simulink model "PVFarmDistributionSystem"  (R2022b)
settings: Solver=FixedStepDiscrete  StartTime=0.0  StopTime=0.6  FixedStep=Ts_Power  RelTol=1e-4
PreLoadFcn:
  | Ts_Power=1e-6;
  | Ts=25e-6;
undefined symbols (not defined in the file): D1, Delta, DiscIntNeverNeededParam, Ion, Lithium
libraries: spsSeriesRLCBranchLib x10, simulink x8, spsMeanLib x5, spsFirstOrderFilterLib x4, spsStairGeneratorLib x4, spsThreePhaseVIMeasurementLib x3, spsPWMGeneratorDCDCLib x3, spsThreePhaseTransformerTwoWindingsLib x2, spsThreePhaseParallelRLCLoadLib x2, spsThreePhasePISectionLineLib x2, spsBoostConverterLib x2, spsPowerPositiveSequenceLib x2
(part 1 of 2)
settings Model: SimulationMode=accelerator  Creator=The MathWorks, Inc.  LastModifiedBy=刘明炜
settings SolverCC: AlgebraicLoopSolver=TrustRegion
settings DataIOCC: SaveOutput=off  SignalLogging=off  DSMLogging=off  SaveTime=off  ReturnWorkspaceOutputs=off
settings OptimizationCC: ReuseModelBlockBuffer=on
settings DebuggingCC: UnconnectedInputMsg=warning  UnconnectedOutputMsg=warning  UnconnectedLineMsg=warning  ArithmeticOperatorsInVariantConditions=warning
settings ModelReferenceCC: EnableRefExpFcnMdlSchedulingChecks=on
settings SFSimCC: CustomCodeUndefinedFunction=UseInterfaceOnly

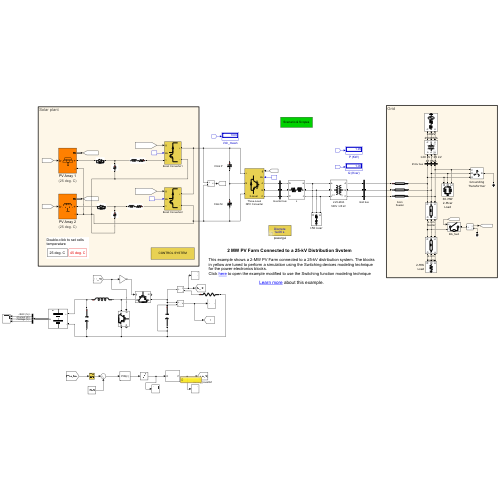
[thumbnail: Simulink's stored preview of the top-level diagram]
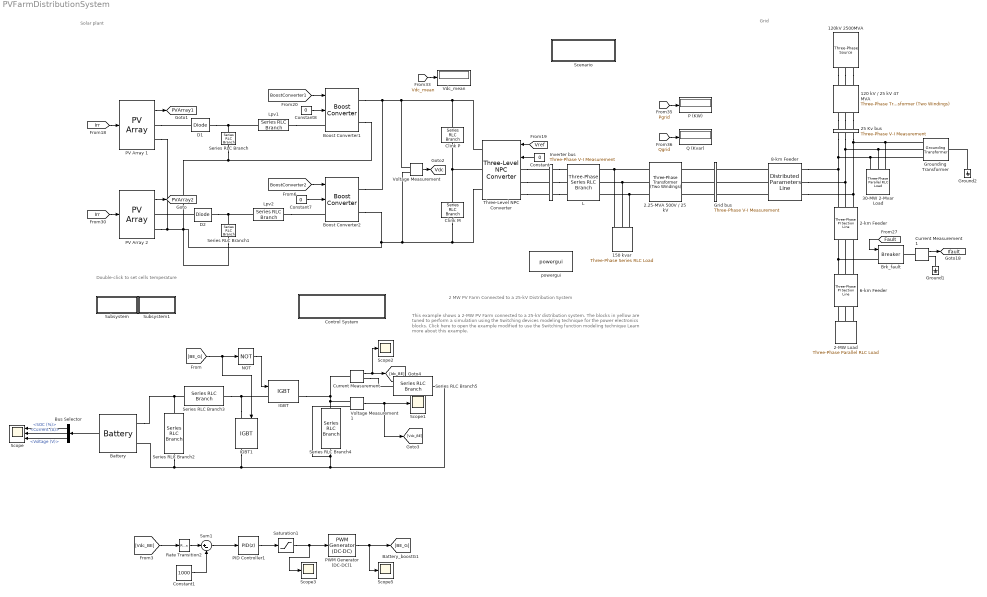
== system PVFarmDistributionSystem ==
  note: Grid
  note: Solar plant
  note: Double-click to set cells temperature
  note: 2 MW PV Farm Connected to a 25-kV Distribution System
  note: This example shows a 2-MW PV Farm connected to a 25-kV distribution system. The blocks in yellow are tuned to perform a simulation using the Switching devices modeling technique for the power electronics blocks.
      | Click here to open the example modified to use the Switching function modeling technique
      |
      | Learn more about this example.
  120 kV / 25 kV 47 MVA : spsThreePhaseTransformerTwoWindingsLib/Three-Phase Transformer (Two Windings)  Winding1Connection=Yg  Winding2Connection=Delta (D1)  CoreType=Three single-phase transformers  SetSaturation=off  Hysteresis=off  DataFile='basic_model'  SetInitialFlux=off  Measurements=None  UNITS=pu  NominalPower=[47e6 50 ]  Winding1="[ 120e3  0.08/30   0.08 ]"  Winding2="[ 25e3 0.08/30  0.08]"  Rm=500  Lm=500  L0=0.5  Saturation="[ 0,0  ;  0.005,1.2  ;  1.0,1.4 ]"  InitialFluxes=[ 0.8 , -0.8 , 0.7 ]  BreakLoop=off  DiscreteSolver=Trapezoidal iterative  DataType=off  TransfoNumber=0
  120kV 2500MVA : spsThreePhaseSourceLib/Three-Phase Source  InternalConnection=Yg  VoltagePhases=off  Voltage=120e3*1.02  PhaseAngle=0  Voltage_phases=[25e3 25e3 25e3]/sqrt(3)  PhaseAngles_phases=[0 -120 +120]  Frequency=50  NonIdealSource=on  SpecifyImpedance=on  Resistance=0.8929  Inductance=16.58e-3  ShortCircuitLevel=2500e6  BaseVoltage=120e3  XRratio=7  BusType=swing  Pref=0  Qref=0  Prefabc=[10e3, 10e3, 10e3]  Qrefabc=[0, 0, 0]  Qmin=-inf  Qmax=inf
  150 kvar : spsThreePhaseSeriesRLCLoadLib/Three-Phase Series RLC Load  LConnTagsString=A|B|C  Configuration=Y (grounded)  NominalVoltage=500  Vabc=[1e3 1e3 1e3]  Vabcp=[1e3 1e3 1e3]  NominalFrequency=50  UnbalancedPower=off  ActivePower=150e3/50  InductivePower=0  CapacitivePower=150e3  Pabc=[10e3 9e3 11e3]  QLabc=[100 90 110]  QCabc=[100 90 110]  Pabcp=[10e3 9e3 11e3]  QLabcp=[100 90 110]  QCabcp=[100 90 110]  Measurements=None  LoadType=constant Z
  2-MW Load : spsThreePhaseParallelRLCLoadLib/Three-Phase Parallel RLC Load  LConnTagsString=A|B|C  Configuration=Y (grounded)  NominalVoltage=25e3  Vabc=[1e3 1e3 1e3]  Vabcp=[1e3 1e3 1e3]  NominalFrequency=50  UnbalancedPower=off  ActivePower=2e6  InductivePower=0  CapacitivePower=0  Pabc=[10e3 9e3 11e3]  QLabc=[100 90 110]  QCabc=[100 90 110]  Pabcp=[10e3 9e3 11e3]  QLabcp=[100 90 110]  QCabcp=[100 90 110]  Measurements=None  LoadType=constant Z
  2-km Feeder : spsThreePhasePISectionLineLib/Three-Phase PI Section Line  LConnTagsString=a|b|c  RConnTagsString=A|B|C  Length=2  Frequency=50  Resistances=[0.1153 0.413]  Inductances=[1.05e-3 3.32e-3]  Capacitances=[11.33e-009 5.01e-009]
  2.25-MVA 500V / 25 kV : spsThreePhaseTransformerTwoWindingsLib/Three-Phase Transformer (Two Windings)  Winding1Connection=Yg  Winding2Connection=Delta (D1)  CoreType=Three single-phase transformers  SetSaturation=off  Hysteresis=off  DataFile='hysteresis'  SetInitialFlux=off  Measurements=None  UNITS=pu  NominalPower=[2.25e6 , 50 ]  Winding1=[ 25e3 , 0.001 , 0.03 ]  Winding2=[500 , 0.001 , 0.03 ]  Rm=200  Lm=200  L0=0.5  Saturation=[ 0,0 ; 0.0024,1.2 ; 1.0,1.52 ]  InitialFluxes=[ 0.8 , -0.8 , 0.7 ]  BreakLoop=off  DiscreteSolver=Trapezoidal iterative  DataType=off  TransfoNumber=0
  25 Kv bus : spsThreePhaseVIMeasurementLib/Three-Phase V-I Measurement  VoltageMeasurement=phase-to-ground  SetLabelV=on  LabelV=Vabc25kV  Vpu=off  VpuLL=off  CurrentMeasurement=yes  SetLabelI=on  LabelI=Iabc25kV  Ipu=off  Pbase=100e6  Vbase=500e3  OutputType=Complex  PhasorSimulation=off  PSBequivalent=0
  30-MW 2-Mvar Load : spsThreePhaseParallelRLCLoadLib/Three-Phase Parallel RLC Load  LConnTagsString=A|B|C  Configuration=Y (grounded)  NominalVoltage=25e3  Vabc=[1e3 1e3 1e3]  Vabcp=[1e3 1e3 1e3]  NominalFrequency=50  UnbalancedPower=off  ActivePower=30e6  InductivePower=2e6  CapacitivePower=0  Pabc=[10e3 9e3 11e3]  QLabc=[100 90 110]  QCabc=[100 90 110]  Pabcp=[10e3 9e3 11e3]  QLabcp=[100 90 110]  QCabcp=[100 90 110]  Measurements=None  LoadType=constant Z
  6-km Feeder : spsThreePhasePISectionLineLib/Three-Phase PI Section Line  LConnTagsString=a|b|c  RConnTagsString=A|B|C  Length=6  Frequency=50  Resistances=[0.1153 0.413]  Inductances=[1.05e-3 3.32e-3]  Capacitances=[11.33e-009 5.01e-009]
  8-km Feeder : spsDistributedParametersLineLib/Distributed Parameters Line  Phases=3  Length=8  Frequency=50  Resistance=[0.1153 0.413]  Inductance=[1.05e-3 3.32e-3]  Capacitance=[11.33e-009 5.01e-009]  x1=[-3.3e-05 -0.0265033347341034 -3248.46958209552 -24803.9467011839;-3.2e-05 -0.0265134091291118 -3240.67704414589 -24804.9660112368;-3.1e-05 -0.0265234809073516 -3232.88418635427 -24805.9828731378;-3e-05 -0.0265335500678288 -3225.09100948977 -24806.9972867864;-2.9e-05 -0.0265436166095496 -3217.29751432154 -24808.0092520825;-2.8e-05 -0.0265536805315205 -3209.50370161879 -24809.0187689262;-2.7e-05 -0.0265637418327481 -3201.70957215071 -24810.025837218;-2.6e-05 -0.0265738005122396 -3193.91512668657 -24811.0304568584;-2.5e-05 -0.026583856569002 -3186.12036599565 -24812.0326277483;-2.4e-05 -0.0265939100020431 -3178.32529084725 -24813.0323497887;-2.3e-05 -0.0266039608103704 -3170.52990201072 -24814.029622881;-2.2e-05 -0.0266140089929921 -3162.73420025543 -24815.0244469268;-2.1e-05 -0.0266240545489164 -3154.9381863508 -24816.0168218278;-2e-05 -0.0266340974771518 -3147.14186106624 -24817.0067474862;-1.9e-05 -0.0266441377767072 -3139.34522517124 -24817.9942238042;-1.8e-05 -0.0266541754465917 -3131.54827943529 -24818.9792506844;-1.7e-05 -0.0266642104858145 -3123.75102462791 -24819.9618280295;-1.6e-05 -0.0266742428933852 -3115.95346151867 -24820.9419557426;-1.5e-05 -0.0266842726683137 -3108.15559087715 -24821.9196337269;-1.4e-05 -0.0266942998096101 -3100.35741347297 -24822.894861886;-1.3e-05 -0.0267043243162847 -3092.55893007578 -24823.8676401236;-1.2e-05 -0.0267143461873481 -3084.76014145526 -24824.8379683437;-1.1e-05 -0.0267243654218113 -3076.96104838112 -24825.8058464505;-1e-05 -0.0267343820186854 -3069.1616516231 -24826.7712743485;-9e-06 -0.0267443959769817 -3061.36195195097 -24827.7342519424;-8e-06 -0.026754407295712 -3053.56195013453 -24828.6947791371;-7e-06 -0.0267644159738881 -3045.76164694361 -24829.652855838;-6e-06 -0.0267744220105223 -3037.96104314806 -24830.6084819503;-5e-06 -0.026784425404627 -3030.16013951778 -24831.5616573798;-4e-06 -0.0267944261552148 -3022.35893682268 -24832.5123820325;-3e-06 -0.0268044242612989 -3014.55743583272 -24833.4606558144;-2e-06 -0.0268144197218923 -3006.75563731786 -24834.406478632;-1e-06 -0.0268244125360086 -2998.95354204812 -24835.349850392]  x2=[-3.3e-05 -0.0341174630392466 -3239.57935848666 -24789.8574696466;-3.2e-05 -0.0341341517787849 -3231.79124723035 -24790.8739874471;-3.1e-05 -0.0341508371494174 -3224.00281700904 -24791.8880584864;-3e-05 -0.0341675191494974 -3216.2140685914 -24792.8996826644;-2.9e-05 -0.0341841977773784 -3208.42500274616 -24793.9088598814;-2.8e-05 -0.0342008730314144 -3200.63562024207 -24794.9155900376;-2.7e-05 -0.0342175449099596 -3192.8459218479 -24795.9198730338;-2.6e-05 -0.0342342134113685 -3185.05590833248 -24796.9217087708;-2.5e-05 -0.0342508785339959 -3177.26558046464 -24797.9210971498;-2.4e-05 -0.0342675402761972 -3169.47493901326 -24798.9180380721;-2.3e-05 -0.0342841986363279 -3161.68398474725 -24799.9125314392;-2.2e-05 -0.0343008536127438 -3153.89271843553 -24800.9045771532;-2.1e-05 -0.0343175052038011 -3146.10114084709 -24801.894175116;-2e-05 -0.0343341534078565 -3138.30925275091 -24802.8813252299;-1.9e-05 -0.0343507982232668 -3130.51705491602 -24803.8660273977;-1.8e-05 -0.0343674396483892 -3122.72454811149 -24804.848281522;-1.7e-05 -0.0343840776815814 -3114.9317331064 -24805.8280875059;-1.6e-05 -0.0344007123212011 -3107.13861066987 -24806.8054452527;-1.5e-05 -0.0344173435656066 -3099.34518157106 -24807.780354666;-1.4e-05 -0.0344339714131565 -3091.55144657914 -24808.7528156495;-1.3e-05 -0.0344505958622096 -3083.75740646333 -24809.7228281073;-1.2e-05 -0.0344672169111253 -3075.96306199286 -24810.6903919437;-1.1e-05 -0.034483834558263 -3068.16841393701 -24811.655507063;-1e-05 -0.0345004488019827 -3060.37346306507 -24812.6181733701;-9e-06 -0.0345170596406447 -3052.57821014639 -24813.57839077;-8e-06 -0.0345336670726094 -3044.78265595031 -24814.5361591679;-7e-06 -0.0345502710962378 -3036.98680124624 -24815.4914784692;-6e-06 -0.0345668717098912 -3029.19064680358 -24816.4443485798;-5e-06 -0.0345834689119311 -3021.39419339179 -24817.3947694054;-4e-06 -0.0346000627007194 -3013.59744178035 -24818.3427408524;-3e-06 -0.0346166530746185 -3005.80039273877 -24819.2882628272;-2e-06 -0.0346332400319909 -2998.00304703658 -24820.2313352364;-1e-06 -0.0346498235711995 -2990.20540544335 -24821.171957987]  x3=[-3.3e-05 0.0018330109452432 -5.20094376290719 -82.5841573333767;-3.2e-05 0.00183248033431178 -5.17499896715227 -82.5857871710245;-3.1e-05 0.00183194954252181 -5.14905366064543 -82.587408857782;-3e-05 0.00183141856992567 -5.12310784594737 -82.589022393489;-2.9e-05 0.00183088741657575 -5.09716152561884 -82.5906277779862;-2.8e-05 0.0018303560825245 -5.07121470222063 -82.5922250111153;-2.7e-05 0.00182982456782434 -5.0452673783136 -82.5938140927186;-2.6e-05 0.00182929287252774 -5.01931955645864 -82.5953950226393;-2.5e-05 0.00182876099668717 -4.9933712392167 -82.5969678007212;-2.4e-05 0.00182822894035512 -4.96742242914877 -82.5985324268093;-2.3e-05 0.00182769670358412 -4.94147312881591 -82.600088900749;-2.2e-05 0.00182716428642668 -4.9155233407792 -82.6016372223868;-2.1e-05 0.00182663168893535 -4.88957306759979 -82.6031773915699;-2e-05 0.0018260989111627 -4.86362231183886 -82.6047094081462;-1.9e-05 0.00182556595316132 -4.83767107605766 -82.6062332719645;-1.8e-05 0.0018250328149838 -4.81171936281746 -82.6077489828744;-1.7e-05 0.00182449949668277 -4.7857671746796 -82.6092565407264;-1.6e-05 0.00182396599831085 -4.75981451420545 -82.6107559453717;-1.5e-05 0.0018234323199207 -4.73386138395645 -82.6122471966622;-1.4e-05 0.00182289846156501 -4.70790778649406 -82.6137302944507;-1.3e-05 0.00182236442329644 -4.6819537243798 -82.615205238591;-1.2e-05 0.00182183020516772 -4.65599920017523 -82.6166720289374;-1.1e-05 0.00182129580723156 -4.63004421644197 -82.6181306653452;-1e-05 0.00182076122954072 -4.60408877574165 -82.6195811476704;-9e-06 0.00182022647214794 -4.578132880636 -82.6210234757698;-8e-06 0.00181969153510602 -4.55217653368674 -82.6224576495012;-7e-06 0.00181915641846774 -4.52621973745568 -82.6238836687229;-6e-06 0.00181862112228592 -4.50026249450463 -82.6253015332942;-5e-06 0.00181808564661339 -4.47430480739548 -82.6267112430751;-4e-06 0.00181754999150301 -4.44834667869016 -82.6281127979266;-3e-06 0.00181701415700763 -4.42238811095061 -82.6295061977104;-2e-06 0.00181647814318014 -4.39642910673886 -82.6308914422888;-1e-06 0.00181594195007344 -4.37046966861695 -82.6322685315251]  x4=[-3.3e-05 -0.00190671763640625 -16.7682219944814 -79.863855689428;-3.2e-05 -0.00190621992184286 -16.743131236574 -79.8691196346437;-3.1e-05 -0.0019057220191431 -16.7180388261858 -79.8743756970934;-3e-05 -0.00190522392835613 -16.6929447657932 -79.8796238762582;-2.9e-05 -0.00190472564953108 -16.6678490578731 -79.8848641716203;-2.8e-05 -0.00190422718271716 -16.6427517049023 -79.8900965826623;-2.7e-05 -0.00190372852796354 -16.6176527093577 -79.8953211088679;-2.6e-05 -0.00190322968531946 -16.5925520737165 -79.9005377497214;-2.5e-05 -0.00190273065483413 -16.5674498004561 -79.905746504708;-2.4e-05 -0.00190223143655682 -16.542345892054 -79.9109473733137;-2.3e-05 -0.00190173203053679 -16.5172403509877 -79.916140355025;-2.2e-05 -0.00190123243682333 -16.4921331797352 -79.9213254493294;-2.1e-05 -0.00190073265546575 -16.4670243807744 -79.9265026557153;-2e-05 -0.00190023268651339 -16.4419139565835 -79.9316719736716;-1.9e-05 -0.00189973253001557 -16.4168019096407 -79.9368334026881;-1.8e-05 -0.00189923218602167 -16.3916882424245 -79.9419869422555;-1.7e-05 -0.00189873165458107 -16.3665729574136 -79.9471325918651;-1.6e-05 -0.00189823093574317 -16.3414560570866 -79.9522703510091;-1.5e-05 -0.00189773002955739 -16.3163375439227 -79.9574002191803;-1.4e-05 -0.00189722893607316 -16.2912174204007 -79.9625221958725;-1.3e-05 -0.00189672765533994 -16.2660956890001 -79.9676362805801;-1.2e-05 -0.00189622618740721 -16.2409723522001 -79.9727424727985;-1.1e-05 -0.00189572453232445 -16.2158474124805 -79.9778407720236;-1e-05 -0.00189522269014119 -16.1907208723209 -79.9829311777523;-9e-06 -0.00189472066090694 -16.1655927342012 -79.9880136894821;-8e-06 -0.00189421844467126 -16.1404630006014 -79.9930883067115;-7e-06 -0.00189371604148372 -16.1153316740019 -79.9981550289396;-6e-06 -0.0018932134513939 -16.0901987568828 -80.0032138556663;-5e-06 -0.0018927106744514 -16.0650642517248 -80.0082647863924;-4e-06 -0.00189220771070584 -16.0399281610085 -80.0133078206194;-3e-06 -0.00189170456020688 -16.0147904872148 -80.0183429578494;-2e-06 -0.00189120122300415 -15.9896512328247 -80.0233701975856;-1e-06 -0.00189069769914735 -15.9645104003192 -80.0283895393318]  x5=3.26270562570392e-05  V1=ones(3,3)  V2=ones(3,3)  I1=ones(3,3)  I2=ones(3,3)  nHarmo=1  Measurements=None  Decoupling=off  VsMag0=0  VrMag0=0  VsAngle0=0  VrAngle0=0  IsMag0=0  IrMag0=0  IsAngle0=0  IrAngle0=0
      settings: LibrarySourceBlock=sps_lib/Power Grid Elements/Distributed Parameters Line
  Battery : spsBatteryLib/Battery  BatType=Lithium-Ion  ShowTempParam=off  ThermalPreset=no  ShowAgeParam=off  NomV=300  NomQ=100  SOC=70  Batt_Tr=1  PresetModel=on  MaxQ=100  MinV=225  FullV=349.1961  Dis_rate=43.4783  R=0.03  Normal_OP=90.4348  expZone="[324.1158      4.913043]"  current=[6.5 13 32.5]  Units=Time  Tci=20  NomT=20  T2=-30  MaxQ2=4.8  FullV2=7.1  Normal_OP2=5.655  expZone2="[6.58           1]"  Rca=0.6  ti=2000  Dp=0  Neq0=0  Tsim=1e6  Ta1=25  Qeol=5.4*0.9  Reol=0.013333*1.2  Char_age=[2.3478, 3]  Dis_age=[2.3478, 10]  N1=1500  N2=10500  N3=1000  N4=1400  Ta2=45  N5=950
  Boost Converter1 : spsBoostConverterLib/Boost Converter  ModelType=Switching devices  Ron=1e-4  Rs=1e6  Cs=inf  Vforward=[0,0]  Ron_Diode=1e-4  Rs_Diode=1e6  Cs_Diode=inf  Vf_Diode=0  Rs_CurrentSource=inf  Ron_ACsource=1e-3
      settings: LibrarySourceBlock=sps_lib/Power Electronics/Boost Converter
  Boost Converter2 : spsBoostConverterLib/Boost Converter  ModelType=Switching devices  Ron=1e-4  Rs=1e6  Cs=inf  Vforward=[0,0]  Ron_Diode=1e-4  Rs_Diode=1e6  Cs_Diode=inf  Vf_Diode=0  Rs_CurrentSource=inf  Ron_ACsource=1e-3
      settings: LibrarySourceBlock=sps_lib/Power Electronics/Boost Converter
  Brk_fault : spsBreakerLib/Breaker  InitialState=0  SwitchingTimes="[30/60  42/60]*999"  External=on  BreakerResistance=0.2  SnubberResistance=1e6  SnubberCapacitance=inf  Measurements=None  MoreParameters=on  NoBreakLoop=off
  Bus Selector : BusSelector  OutputSignals=SOC (%),Current (A),Voltage (V)
  Clink M : spsSeriesRLCBranchLib/Series RLC Branch  LConnTagsString=__new0  RConnTagsString=__new0  BranchType=C  Resistance=1e-6  Inductance=1e-3  SetiL0=off  InitialCurrent=0  Capacitance=150e-3  Setx0=on  InitialVoltage=500  Measurements=None
  Clink P : spsSeriesRLCBranchLib/Series RLC Branch  LConnTagsString=__new0  RConnTagsString=__new0  BranchType=C  Resistance=1e-6  Inductance=1e-3  SetiL0=off  InitialCurrent=0  Capacitance=150e-3  Setx0=on  InitialVoltage=500  Measurements=None
  Constant : Constant  Value=0  SampleTime=Ts
  Constant1 : Constant  Value=1000
  Constant7 : Constant  Value=0  SampleTime=Ts
  Constant8 : Constant  Value=0  SampleTime=Ts
  Control System : Subsystem
      mask Display: disp('CONTROL SYSTEM')
  Current Measurement : spsCurrentMeasurementLib/Current Measurement  PhasorSimulation=off  OutputType=Complex  PSBequivalent=0
  Current Measurement1 : spsCurrentMeasurementLib/Current Measurement  PhasorSimulation=off  OutputType=Complex  PSBequivalent=0
  D1 : spsDiodeLib/Diode  Ron=1e-4  Lon=0  Vf=0  IC=0  UseSnubber=0  Rs=1e6  Cs=inf  Measurements=off
  D2 : spsDiodeLib/Diode  Ron=1e-4  Lon=0  Vf=0  IC=0  UseSnubber=0  Rs=1e6  Cs=inf  Measurements=off
  Grid bus : spsThreePhaseVIMeasurementLib/Three-Phase V-I Measurement  VoltageMeasurement=phase-to-ground  SetLabelV=on  LabelV=Vgrid  Vpu=off  VpuLL=off  CurrentMeasurement=yes  SetLabelI=on  LabelI=Igrid  Ipu=off  Pbase=100e6  Vbase=500e3  OutputType=Magnitude  PhasorSimulation=off  PSBequivalent=0
  Ground1 : spsGroundLib/Ground  LConnTagsString=a
  Ground2 : spsGroundLib/Ground  LConnTagsString=a
  Grounding Transformer : spsGroundingTransformerLib/Grounding Transformer   UNITS=SI  NominalPower="[3e6   50]"  NominalVoltage=25e3  ZeroSequenceImpedance_pu=[0.0012 0.036]  MagnetizationBranch_pu=[500 500]  ZeroSequenceImpedance_SI=[0.25 7.5]  MagnetizationBranch_SI=[1.0417e+05 1.0417e+05]  Measurements=None
      settings: LibrarySourceBlock=|
      | sps_lib/Power Grid Elements/Grounding
      | Transformer
  IGBT : spsIGBTLib/IGBT  Ron=0.001  Lon=0  Vf=1  Tf=1e-6  Tt=2e-6  IC=0  Rs=1e5  Cs=inf  Measurements=on
  IGBT1 : spsIGBTLib/IGBT  Ron=0.001  Lon=0  Vf=1  Tf=1e-6  Tt=2e-6  IC=0  Rs=1e5  Cs=inf  Measurements=on
  Inverter bus : spsThreePhaseVIMeasurementLib/Three-Phase V-I Measurement  VoltageMeasurement=phase-to-phase  SetLabelV=on  LabelV=Vinv  Vpu=off  VpuLL=off  CurrentMeasurement=no  SetLabelI=off  LabelI=Iabc_B1  Ipu=off  Pbase=100e6  Vbase=500e3  OutputType=Magnitude  PhasorSimulation=off  PSBequivalent=0
  L : spsThreePhaseSeriesRLCBranchLib/Three-Phase Series RLC Branch  LConnTagsString=A|B|C  RConnTagsString=A|B|C  BranchType=RL  Resistance=1e-3  Inductance=44.2e-6  Capacitance=inf  Measurements=None
  Lpv1 : spsSeriesRLCBranchLib/Series RLC Branch  LConnTagsString=__new0  RConnTagsString=__new0  BranchType=RL  Resistance=1e-3  Inductance=1e-3  SetiL0=off  InitialCurrent=0  Capacitance=120e-3  Setx0=off  InitialVoltage=0  Measurements=None
  Lpv2 : spsSeriesRLCBranchLib/Series RLC Branch  LConnTagsString=__new0  RConnTagsString=__new0  BranchType=RL  Resistance=1e-3  Inductance=1e-3  SetiL0=off  InitialCurrent=0  Capacitance=120e-3  Setx0=off  InitialVoltage=0  Measurements=None
  NOT : Logic  Operator=NOT  IconShape=distinctive  AllPortsSameDT=off  OutDataTypeStr=boolean
  P (KW) : Display
      settings: Format=bank  Decimation=200
  PID Controller1 : slpidlib/PID Controller  Controller=PID  Form=Parallel  TimeDomain=Discrete-time  UseExternalTs=off  SampleTime=-1  IntegratorMethod=Forward Euler  FilterMethod=Forward Euler  ControllerParametersSource=internal  P=1  I=1  UseKiTs=off  D=0  N=100  UseFilter=on  TunerSelectOption=Transfer Function Based (PID Tuner App)  InitialConditionSource=internal  InitialConditionForIntegrator=0  InitialConditionForFilter=0  DifferentiatorICPrevScaledInput=0  ExternalReset=none  TrackingMode=off  Kt=1  LimitOutput=off  SatLimitsSource=internal  UpperSaturationLimit=0.99  LowerSaturationLimit=0.1  LinearizeAsGain=on  AntiWindupMode=none  Kb=1  LimitIntegrator=off  UpperIntegratorSaturationLimit=inf  LowerIntegratorSaturationLimit=-inf  POutMin=[]  POutMax=[]  IOutMin=[]  IOutMax=[]  DOutMin=[]  DOutMax=[]  NOutMin=[]  NOutMax=[]  SumOutMin=[]  SumOutMax=[]  SaturationOutMin=[]  SaturationOutMax=[]  PParamMin=[]  PParamMax=[]  IParamMin=[]  IParamMax=[]  DParamMin=[]  DParamMax=[]  NParamMin=[]  NParamMax=[]  KbParamMin=[]  KbParamMax=[]  KtParamMin=[]  KtParamMax=[]  KbOutMin=[]  KbOutMax=[]  KtOutMin=[]  KtOutMax=[]  IntegratorOutMin=[]  IntegratorOutMax=[]  FilterOutMin=[]  FilterOutMax=[]  SumI1OutMin=[]  SumI1OutMax=[]  SumI2OutMin=[]  SumI2OutMax=[]  SumI3OutMin=[]  SumI3OutMax=[]  SumI4OutMin=[]  SumI4OutMax=[]  SumDOutMin=[]  SumDOutMax=[]  DifferentiatorOutMin=[]  DifferentiatorOutMax=[]  FilterDiffOutCoefMin=[]  FilterDiffOutCoefMax=[]  ReciprocalOutMin=[]  ReciprocalOutMax=[]  SumDenOutMin=[]  SumDenOutMax=[]  SumNumOutMin=[]  SumNumOutMax=[]  DivideOutMin=[]  DivideOutMax=[]  UdiffTsProdOutMin=[]  UdiffTsProdOutMax=[]  NTsProdOutMin=[]  NTsProdOutMax=[]  UintegralTsProdOutMin=[]  UintegralTsProdOutMax=[]  UngainTsProdOutMin=[]  UngainTsProdOutMax=[]  ClampingZeroOutDataTypeStr=Inherit: Inherit via back propagation  ClampingZeroOutMin=[]  ClampingZeroOutMax=[]  FilterDenConstantOutDataTypeStr=Inherit: Inherit via back propagation  FilterDenConstantOutMin=[]  FilterDenConstantOutMax=[]  PCopyOutDataTypeStr=Inherit: Inherit via back propagation  PCopyOutMin=[]  PCopyOutMax=[]  NCopyOutDataTypeStr=Inherit: Inherit via back propagation  NCopyOutMin=[]  NCopyOutMax=[]  IntegratorContinuousStateAttributes=''  IntegratorStateMustResolveToSignalObject=off  IntegratorRTWStateStorageClass=Auto  FilterContinuousStateAttributes=''  FilterStateMustResolveToSignalObject=off  FilterRTWStateStorageClass=Auto  ParallelPVariant=InternalParameters  IdealPVariant=Disabled  IVariant=InternalParameters  DVariant=InternalParameters  IntegratorVariant=Discrete  SatVariant=Disabled  AWVariant=Passthrough  PCopyVariant=Disabled  TRVariant=Disabled  FdbkBlocksVariant=Forward  IdealPFdbkVariant=Disabled  SatFdbkVariant=Disabled  DerivativeFilterVariant=ForwardEulerFilter  NVariant=InternalParameters  NCopyVariant=Disabled  FilterICVariant=InternalICsFilter  IntegratorICVariant=InternalICs  ExternalResetVariant=Disabled  TRSumVariant=Passthrough  SumFdbkVariant=Disabled  SumVariant=Sum_PID  TsampFilterVariant=InternalTs  TsampNgainVariant=Passthrough  TsampIntegralVariant=Passthrough  ExternalSaturationOutDataTypeStr=Inherit: Same as second input
  PV Array 1 : spsPVArrayLib/PV Array  Npar=282  Nser=15  PlotType=array @ 1000 W/m2 & specified temperatures  S_vec=[ 1000 250]  Temp_C_vec="[ 45 25  ]"  ModuleName=User-defined  PlotWhenSelected=off  Pm=355.012  Ncell=83  Voc=51.9  Isc=8.68  Vm=43.4  Im=8.18  beta_Voc_pc=-0.304  alpha_Isc_pc=0.017  beta_Voc=-0.15778  alpha_Isc=0.0014756  IL=8.6865  I0=3.3093e-11  nI=0.92618  Rsh=389.4331  Rs=0.29289  RobustModel=on  RobustCellTemperature=25  BAL=on  Tc=1e-6  Tfilter=5e-5
      settings: AttributesFormatString=(%<RobustCellTemperature> deg. C)
  PV Array 2 : spsPVArrayLib/PV Array  Npar=122  Nser=14  PlotType=array @ 1000 W/m2 & specified temperatures  S_vec=[ 1000 250]  Temp_C_vec="[ 45 25  ]"  ModuleName=User-defined  PlotWhenSelected=off  Pm=293.664  Ncell=60  Voc=39.5  Isc=9.60  Vm=32.2  Im=9.12  beta_Voc_pc=-0.300  alpha_Isc_pc=0.03  beta_Voc=-0.1185  alpha_Isc=0.00288  IL=9.6627  I0=3.1923e-11  nI=0.96973  Rsh=336.4947  Rs=0.3029  RobustModel=on  RobustCellTemperature=25  BAL=on  Tc=1e-6  Tfilter=5e-5
      settings: AttributesFormatString=(%<RobustCellTemperature> deg. C)
  PWM Generator (DC-DC)1 : spsPWMGeneratorDCDCLib/PWM Generator (DC-DC)  Fsw=10000  Ts=0
  Q (Kvar) : Display
      settings: Format=bank  Decimation=200
  Rate Transition2 : RateTransition  OutPortSampleTime=Ts
  Saturation1 : Saturate  UpperLimit=0.99  LowerLimit=0.01
  Scenario : Subsystem
      mask Display: disp('Scenario & Scopes')
  Scope : Scope  NumInputPorts=3
  Scope{1..3,5} (4 alike) : Scope
  Series RLC Branch : spsSeriesRLCBranchLib/Series RLC Branch  LConnTagsString=__new0  RConnTagsString=__new0  BranchType=C  Resistance=1  Inductance=1e-3  SetiL0=off  InitialCurrent=0  Capacitance=200e-6  Setx0=on  InitialVoltage=650  Measurements=None
  Series RLC Branch1 : spsSeriesRLCBranchLib/Series RLC Branch  LConnTagsString=__new0  RConnTagsString=__new0  BranchType=C  Resistance=1  Inductance=1e-3  SetiL0=off  InitialCurrent=0  Capacitance=200e-6  Setx0=on  InitialVoltage=450  Measurements=None
  Series RLC Branch2 : spsSeriesRLCBranchLib/Series RLC Branch  LConnTagsString=__new0  RConnTagsString=__new0  BranchType=C  Resistance=1  Inductance=1e-3  SetiL0=off  InitialCurrent=0  Capacitance=470e-6  Setx0=off  InitialVoltage=0  Measurements=None
  Series RLC Branch3 : spsSeriesRLCBranchLib/Series RLC Branch  LConnTagsString=__new0  RConnTagsString=__new0  BranchType=L  Resistance=1  Inductance=2e-3  SetiL0=off  InitialCurrent=0  Capacitance=1e-6  Setx0=off  InitialVoltage=0  Measurements=None
  Series RLC Branch4 : spsSeriesRLCBranchLib/Series RLC Branch  LConnTagsString=__new0  RConnTagsString=__new0  BranchType=C  Resistance=1  Inductance=1e-3  SetiL0=off  InitialCurrent=0  Capacitance=470e-6  Setx0=off  InitialVoltage=0  Measurements=None
  Series RLC Branch5 : spsSeriesRLCBranchLib/Series RLC Branch  LConnTagsString=__new0  RConnTagsString=__new0  BranchType=R  Resistance=10  Inductance=2e-3  SetiL0=off  InitialCurrent=0  Capacitance=1e-6  Setx0=off  InitialVoltage=0  Measurements=None
  Subsystem : Subsystem
      settings: OpenFcn=|
      | SystemName1=gcs;
      | BlockName1=[SystemName1, '/', 'PV Array 1'];
      | set_param(BlockName1,'RobustCellTemperature','25');
      | set_param(BlockName1,'ForegroundColor','black');
      | BlockName2=[SystemName1, '/', 'PV Array 2'];
      | set_param(BlockName2,'RobustCellTemperature','25');
      | set_param(BlockName2,'ForegroundColor','black');
      mask Display: disp('25 deg. C')
  Subsystem1 : Subsystem
      settings: OpenFcn=|
      | SystemName1=gcs;
      | BlockName1=[SystemName1, '/', 'PV Array 1'];
      | set_param(BlockName1,'RobustCellTemperature','45');
      | set_param(BlockName1,'ForegroundColor','red');
      | BlockName2=[SystemName1, '/', 'PV Array 2'];
      | set_param(BlockName2,'RobustCellTemperature','45');
      | set_param(BlockName2,'ForegroundColor','red');
      mask Display: disp('45 deg. C')
  Sum1 : Sum  Inputs=|+-
  Three-Level NPC Converter : spsThreeLevelNPCConverterLib/Three-Level NPC Converter  ModelType=Switching devices  Ron=1e-4/2  Rs=1e6  Cs=inf  Vforward=[0,0]  Ron_Diode=1e-4  Rs_Diode=1e6  Cs_Diode=inf  Vf_Diode=0  Rs_CurrentSource=inf  Ron_ACsource=1e-3
      settings: LibrarySourceBlock=|
      | sps_lib/Power Electronics/Three-Level
      | NPC Converter
  Vdc_mean : Display
      settings: Decimation=200
  Voltage Measurement : spsVoltageMeasurementLib/Voltage Measurement  PhasorSimulation=off  OutputType=Complex  PSBequivalent=0
  Voltage Measurement1 : spsVoltageMeasurementLib/Voltage Measurement  PhasorSimulation=off  OutputType=Complex  PSBequivalent=0
  powergui : sps_lib/powergui  Priority=2  SimulationMode=Discrete  SampleTime=Ts_Power  frequency=60  Iterations=50  frequencyindice=0  Pbase=100e6  ErrMax=1e-4  UnitsV=kV  UnitsW=MW  buscounter=0  FunctionMessages=off  echomessages=off  EnableUseOfTLC=off  CurrentSourceSwitches=off  DisableSnubberDevices=off  DisableRonSwitches=off  DisableVfSwitches=off  DisplayEquations=off  AutomaticDiscreteSolvers=off  SolverType=Tustin/Backward Euler (TBE)  Interpol=off  ExternalGateDelay=off  methode=off  Ts=0  x0status=blocks  SPID=off  SwTol=0  HookPort=off  NonlinearTolerance=1e-4  nMaxIteration=100  ContinueOnMaxIteration=on  RestoreLinks=warning  ResistiveCurrentMeasurement=off  Frange=[0:2:500]  Ylog=off  Xlog=off  ShowGrid=off  save=off  variable=ZData  structure=Scope_VIgrid  ZoomFFT=off  StartTime=0.18  cycles=1  DisplayStyle=1  fundamental=60  FreqAxis=on  MaxFrequency=3500  frequencyindicesteady=1  RmsSteady=1  display=off
  tag scope: Ifault=global, PVArray1=global, PVArray2=global, Vdc=global
  wires:
  Voltage Measurement/1 -> [Vdc]
  PV Array 1/1 -> [PVArray1]
  Constant/1 -> Three-Level NPC Converter/2
  [Irr] -> PV Array 1/1
  Constant7/1 -> Boost Converter2/2
  PV Array 2/1 -> [PVArray2]
  [Irr] -> PV Array 2/1
  Constant8/1 -> Boost Converter1/2
  Current Measurement1/1 -> [Ifault]
  [Fault] -> Brk_fault/1
  [Vref] -> Three-Level NPC Converter/1
  [Vdc_mean] -> Vdc_mean/1
  [Pgrid] -> P (KW)/1
  [Qgrid] -> Q (Kvar)/1
  [BoostConverter1] -> Boost Converter1/1
  [BoostConverter2] -> Boost Converter2/1
  Battery/1 -> Bus Selector/1
  Bus Selector/1 -> Scope/1  "<SOC (%)>"
  Bus Selector/2 -> Scope/2  "<Current (A)>"
  Bus Selector/3 -> Scope/3  "<Voltage (V)>"
  [BE_G] -> IGBT1/1, NOT/1
  Voltage Measurement1/1 -> [Vdc_BE], Scope1/1
  Current Measurement/1 -> Scope2/1, [Idc_BE]
  Sum1/1 -> PID Controller1/1
  PWM Generator (DC-DC)1/1 -> [BE_G], Scope5/1
  Rate Transition2/1 -> Sum1/1
  [Vdc_BE] -> Rate Transition2/1
  Constant1/1 -> Sum1/2
  PID Controller1/1 -> Saturation1/1
  NOT/1 -> IGBT/1
  Saturation1/1 -> Scope3/1, PWM Generator (DC-DC)1/1
  connections:
  Boost Converter1/RConn1 -- Boost Converter2/RConn1 -- Three-Level NPC Converter/RConn1 -- Clink P/LConn1 -- Voltage Measurement/LConn1
  Lpv2/RConn1 -- D2/RConn1 -- Series RLC Branch1/LConn1
  Lpv1/RConn1 -- D1/RConn1 -- Series RLC Branch/LConn1
  120kV 2500MVA/RConn2 -- 120 kV / 25 kV 47 MVA/LConn2
  Inverter bus/RConn2 -- L/LConn2
  120 kV / 25 kV 47 MVA/RConn3 -- 25 Kv bus/LConn3
  Grid bus/LConn1 -- 2.25-MVA 500V / 25 kV/LConn1
  Inverter bus/RConn3 -- L/LConn3
  Lpv2/LConn1 -- Boost Converter2/LConn1
  Three-Level NPC Converter/LConn3 -- Inverter bus/LConn3
  Grid bus/LConn3 -- 2.25-MVA 500V / 25 kV/LConn3
  120 kV / 25 kV 47 MVA/RConn2 -- 25 Kv bus/LConn2
  120kV 2500MVA/RConn1 -- 120 kV / 25 kV 47 MVA/LConn1
  120 kV / 25 kV 47 MVA/RConn1 -- 25 Kv bus/LConn1
  Inverter bus/RConn1 -- L/LConn1
  Three-Level NPC Converter/LConn1 -- Inverter bus/LConn1
  Three-Level NPC Converter/LConn2 -- Inverter bus/LConn2
  Grid bus/LConn2 -- 2.25-MVA 500V / 25 kV/LConn2
  120kV 2500MVA/RConn3 -- 120 kV / 25 kV 47 MVA/LConn3
  Lpv1/LConn1 -- Boost Converter1/LConn1
  Current Measurement1/RConn1 -- Ground1/LConn1
  Current Measurement1/LConn1 -- Brk_fault/RConn1
  PV Array 1/RConn1 -- D1/LConn1
  D2/LConn1 -- PV Array 2/RConn1
  Series RLC Branch/RConn1 -- Boost Converter1/RConn2 -- Boost Converter2/RConn2 -- Clink M/RConn1 -- Three-Level NPC Converter/RConn3 -- Voltage Measurement/LConn2 -- Series RLC Branch1/RConn1 -- PV Array 2/RConn2 -- PV Array 1/RConn2
  2.25-MVA 500V / 25 kV/RConn2 -- 150 kvar/LConn2 -- L/RConn2
  2.25-MVA 500V / 25 kV/RConn1 -- 150 kvar/LConn1 -- L/RConn1
  2.25-MVA 500V / 25 kV/RConn3 -- 150 kvar/LConn3 -- L/RConn3
  Clink M/LConn1 -- Clink P/RConn1 -- Three-Level NPC Converter/RConn2
  2-MW Load/LConn1 -- 6-km Feeder/RConn1
  2-MW Load/LConn2 -- 6-km Feeder/RConn2
  2-MW Load/LConn3 -- 6-km Feeder/RConn3
  6-km Feeder/LConn1 -- Brk_fault/LConn1 -- 2-km Feeder/RConn1
  6-km Feeder/LConn2 -- 2-km Feeder/RConn2
  6-km Feeder/LConn3 -- 2-km Feeder/RConn3
  8-km Feeder/LConn1 -- Grid bus/RConn1
  8-km Feeder/LConn2 -- Grid bus/RConn2
  8-km Feeder/LConn3 -- Grid bus/RConn3
  25 Kv bus/RConn1 -- Grounding Transformer/LConn1 -- 30-MW 2-Mvar Load/LConn1 -- 2-km Feeder/LConn1 -- 8-km Feeder/RConn1
  25 Kv bus/RConn2 -- 2-km Feeder/LConn2 -- 8-km Feeder/RConn2 -- 30-MW 2-Mvar Load/LConn2 -- Grounding Transformer/LConn2
  25 Kv bus/RConn3 -- 30-MW 2-Mvar Load/LConn3 -- Grounding Transformer/LConn3 -- 2-km Feeder/LConn3 -- 8-km Feeder/RConn3
  Ground2/LConn1 -- Grounding Transformer/RConn1
  Battery/LConn1 -- Series RLC Branch3/LConn1 -- Series RLC Branch2/LConn1
  Series RLC Branch2/RConn1 -- Series RLC Branch5/RConn1 -- Voltage Measurement1/LConn2 -- Series RLC Branch4/RConn1 -- IGBT1/RConn1 -- Battery/LConn2
  IGBT1/LConn1 -- IGBT/LConn1 -- Series RLC Branch3/RConn1
  Series RLC Branch4/LConn1 -- Current Measurement/LConn1 -- IGBT/RConn1 -- Voltage Measurement1/LConn1
  Current Measurement/RConn1 -- Series RLC Branch5/LConn1

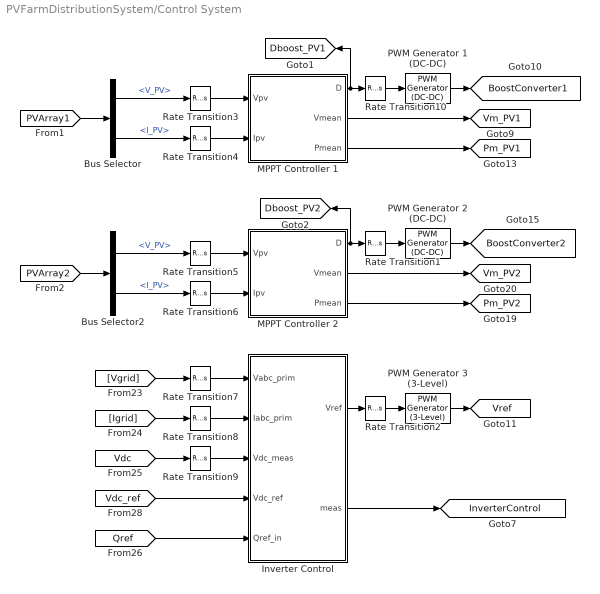
== system PVFarmDistributionSystem/Control System ==
  Bus Selector : BusSelector  OutputSignals=V_PV,I_PV
  Bus Selector2 : BusSelector  OutputSignals=V_PV,I_PV
  Inverter Control : Subsystem  mask(Inverter Control){Pnom=2.25e6, Fnom=50, Vnom_prim=25e3, Vnom_sec=500, Vnom_dc=1000, Kp_Preg=1, Ki_Preg=75, Kp_VDCreg=10, Ki_VDCreg=500, Kp_Ireg=0.3, Ki_Ireg=20, RLff=[ 0.004, 0.21], Ts=Ts}
      mask prompts: Pnom "Power (VA)"; Fnom "Frequency (Hz)"; Vnom_prim "Primary voltage (Vrms)"; Vnom_sec "Secondary voltage (Vrms)"; Vnom_dc "DC voltage (V)"; Kp_Preg "Proportional gain"; Ki_Preg "Integral gain"; Kp_VDCreg "Proportional gain"; Ki_VDCreg "Integral gain"; Kp_Ireg "Proportional gain"; Ki_Ireg "Integral gain"; RLff "Feedforward Values [Rff Lff] (pu)"; Ts "Control sample time:"
      mask help: Control system for a 2-MW, 1-Mvar, 25-kV, Grid-Connected Inverter
      mask init:
      | Rff=RLff(1);
      | Lff=RLff(2);
      | Limits_Ireg=[1.5, -1.5];
      | Limits_VDCreg=[1.5, -1.5];
      | Limits_Preg=[1.5, -1.5];
      | Limits_Qreg=[1.5, -1.5];
      mask DialogControl Container4 Prompt: Nominal Values:
      mask DialogControl Container16 Prompt: Power regulators
      mask DialogControl Container8 Prompt: Voltage regulator:
      mask DialogControl Container6 Prompt: Current regulators:
      mask DialogControl Ts1 Prompt: Sample time (s)
  MPPT Controller 1 : Subsystem  mask(MPPT Controller - Perturb and Observe algorithm (PandO)){Dinit=0.35, Dlimits=[0.8, 0.3], deltaD=60e-6, Fc=1000, Ts=Ts}
      mask prompts: Dinit "Duty cycle (D) initial value"; Dlimits "D limits [Upper, Lower]"; deltaD "Increment value for PandO algorithm"; Fc "Measurement filter cutoff frequency (Hz)"; Ts "Sample time (s)"
      mask init:
      | Dmax=Dlimits(1);
      | Dmin=Dlimits(2);
  MPPT Controller 2 : Subsystem  mask(MPPT Controller - Perturb and Observe algorithm (PandO)){Dinit=0.55, Dlimits=[0.8, 0.47], deltaD=60e-6, Fc=1000, Ts=Ts}
      mask prompts: Dinit "Duty cycle (D) initial value"; Dlimits "D limits [Upper, Lower]"; deltaD "Increment value for PandO algorithm"; Fc "Measurement filter cutoff frequency (Hz)"; Ts "Sample time (s)"
      mask init:
      | Dmax=Dlimits(1);
      | Dmin=Dlimits(2);
  PWM Generator 1 (DC-DC) : spsPWMGeneratorDCDCLib/PWM Generator (DC-DC)  Fsw=5000  Ts=Ts_Power
  PWM Generator 2 (DC-DC) : spsPWMGeneratorDCDCLib/PWM Generator (DC-DC)  Fsw=5000  Ts=Ts_Power
  PWM Generator 3 (3-Level) : spsPWMGenerator3LevelLib/PWM Generator (3-Level)  ModulatorType=Three-phase bridge (12 pulses)  ModulatorMode=Unsynchronized  nF=27  Fc=39*60  ModulatingSignals=off  m=0.8  Freq=60  Phase=0  Ts=Ts_Power
      settings: LibrarySourceBlock=|
      | sps_lib/Power Electronics/Power Electronics Control/PWM Generator
      | (3-Level)
  Rate Transition1 : RateTransition  OutPortSampleTime=Ts_Power
  Rate Transition10 : RateTransition  OutPortSampleTime=Ts_Power
  Rate Transition2 : RateTransition  OutPortSampleTime=Ts_Power
  Rate Transition{3..9} (7 alike) : RateTransition  OutPortSampleTime=Ts
  tag scope: BoostConverter1=global, BoostConverter2=global, Dboost_PV1=global, Dboost_PV2=global, InverterControl=global, Pm_PV1=global, Pm_PV2=global, Vm_PV1=global, Vm_PV2=global, Vref=global
  wires:
  Inverter Control/1(Vref) -> Rate Transition2/1
  MPPT Controller 2/2(Vmean) -> [Vm_PV2]
  [Vgrid] -> Rate Transition7/1
  [Vdc_ref] -> Inverter Control/4(Vdc_ref)
  Bus Selector2/1 -> Rate Transition5/1  "<V_PV>"
  Rate Transition3/1 -> MPPT Controller 1/1(Vpv)
  Rate Transition2/1 -> PWM Generator 3 (3-Level)/1
  Rate Transition4/1 -> MPPT Controller 1/2(Ipv)
  [Igrid] -> Rate Transition8/1
  Bus Selector/2 -> Rate Transition4/1  "<I_PV>"
  MPPT Controller 2/3(Pmean) -> [Pm_PV2]
  [Qref] -> Inverter Control/5(Qref_in)
  [Vdc] -> Rate Transition9/1
  MPPT Controller 1/1(D) -> [Dboost_PV1], Rate Transition10/1
  Bus Selector/1 -> Rate Transition3/1  "<V_PV>"
  Bus Selector2/2 -> Rate Transition6/1  "<I_PV>"
  Rate Transition1/1 -> PWM Generator 2 (DC-DC)/1
  Rate Transition6/1 -> MPPT Controller 2/2(Ipv)
  Rate Transition8/1 -> Inverter Control/2(Iabc_prim)
  Rate Transition7/1 -> Inverter Control/1(Vabc_prim)
  MPPT Controller 1/3(Pmean) -> [Pm_PV1]
  MPPT Controller 1/2(Vmean) -> [Vm_PV1]
  Rate Transition9/1 -> Inverter Control/3(Vdc_meas)
  Rate Transition10/1 -> PWM Generator 1 (DC-DC)/1
  MPPT Controller 2/1(D) -> [Dboost_PV2], Rate Transition1/1
  Rate Transition5/1 -> MPPT Controller 2/1(Vpv)
  PWM Generator 1 (DC-DC)/1 -> [BoostConverter1]
  PWM Generator 2 (DC-DC)/1 -> [BoostConverter2]
  Inverter Control/2(meas) -> [InverterControl]
  PWM Generator 3 (3-Level)/1 -> [Vref]
  [PVArray1] -> Bus Selector/1
  [PVArray2] -> Bus Selector2/1

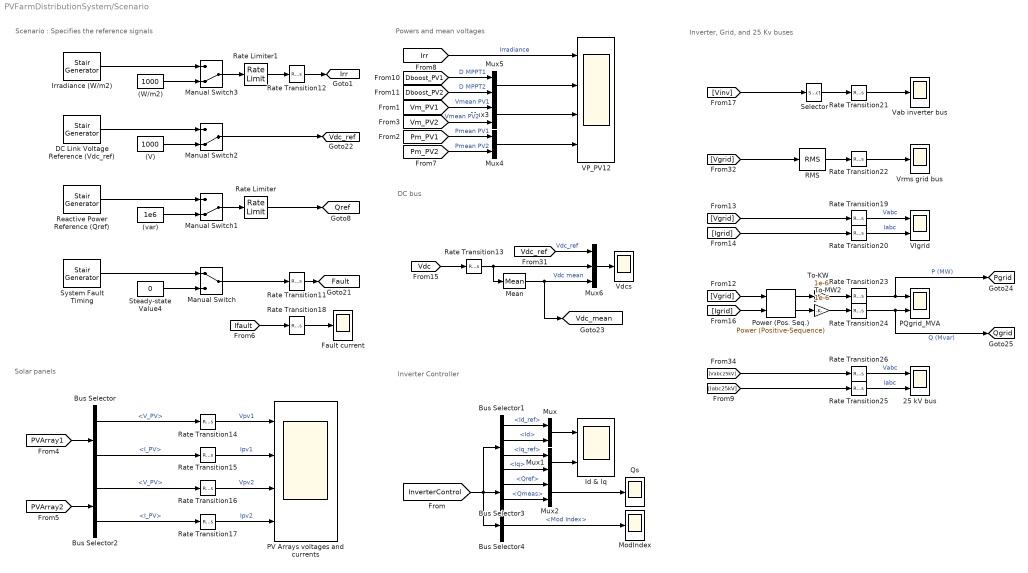
== system PVFarmDistributionSystem/Scenario ==
  note: DC bus
  note: Powers and mean voltages
  note: Inverter, Grid, and 25 Kv buses
  note: Inverter Controller
  note: Solar panels
  note: Scenario : Specifies the reference signals
  (V) : Constant  Value=1000
  (W/m2) : Constant  Value=1000
  (var) : Constant  Value=1e6
  25 kV bus : Scope  NumInputPorts=2
  Bus Selector : BusSelector  OutputSignals=V_PV,I_PV
  Bus Selector1 : BusSelector  OutputSignals=Id_ref,Id,Iq_ref,Iq
  Bus Selector2 : BusSelector  OutputSignals=V_PV,I_PV
  Bus Selector3 : BusSelector  OutputSignals=Qref,Qmeas
  Bus Selector4 : BusSelector  OutputSignals=Mod Index
  DC Link Voltage Reference (Vdc_ref) : spsStairGeneratorLib/Stair Generator  t=[0, 0.2, 0.4]  e=[1000, 1050, 1000]  Ts=Ts
  Fault current : Scope
  Id & Iq : Scope  NumInputPorts=2
  Irradiance (W/m2) : spsStairGeneratorLib/Stair Generator  t=[0, 0.2, 0.4]  e=[1000, 250,1000]  Ts=Ts
  Manual Switch : ManualSwitch
  Manual Switch1 : ManualSwitch  CurrentSetting=0
  Manual Switch2 : ManualSwitch  CurrentSetting=0
  Manual Switch3 : ManualSwitch  CurrentSetting=0
  Mean : spsMeanLib/Mean  Freq=60  Vinit=1000  Ts=Ts
  ModIndex : Scope
  Mux{,1..5} (6 alike) : Mux  Inputs=2
  Mux6 : Mux  Inputs=3
  PQgrid_MVA : Scope  NumInputPorts=2
  PV Arrays voltages and currents : Scope  NumInputPorts=4
  Power (Pos. Seq.) : spsPowerPositiveSequenceLib/Power (Positive-Sequence)  Freq=50  Vinit=[20570,-37]  Iinit=[70, -63]  Ts=Ts_Power
      settings: LibrarySourceBlock=|
      | sps_lib/Sensors and Measurements/Power
      | (Positive-Sequence)
  Qs : Scope
  RMS : spsRMSLib/RMS  TrueRMS=off  Freq=50  RMSInit=25000  Ts=Ts_Power
  Rate Limiter : RateLimiter  RisingSlewLimit=1e6/(1/60)  FallingSlewLimit=-1e6/(1/60)  SampleTimeMode=inherited  InitialCondition=1e6
  Rate Limiter1 : RateLimiter  RisingSlewLimit=1000/(1/60)  FallingSlewLimit=-1000/(1/60)  SampleTimeMode=inherited  InitialCondition=1000
  Rate Transition11 : RateTransition  OutPortSampleTime=Ts_Power
  Rate Transition12 : RateTransition  OutPortSampleTime=Ts_Power
  Rate Transition{13..26} (14 alike) : RateTransition  OutPortSampleTime=Ts
  "Reactive Power Reference (Qref) " : spsStairGeneratorLib/Stair Generator  t=[0, 0.2, 0.4]  e=[1e6, -1e6, 1e6]  Ts=Ts
  Selector : Selector  InputPortWidth=3  IndexOptions=Index vector (dialog)  Indices=1  OutputSizes=1
  Steady-state Value4 : Constant  Value=0
  System Fault Timing : spsStairGeneratorLib/Stair Generator  t=[0, 0.25, 0.45]  e=[0, 1, 0]  Ts=Ts
  To-KW : Gain  Gain=1e-6
  To-MW2 : Gain  Gain=1e-6
  VIgrid : Scope  NumInputPorts=2
  VP_PV12 : Scope  NumInputPorts=4
  Vab inverter bus : Scope
  Vdcs : Scope
  Vrms grid bus : Scope
  tag scope: Fault=global, Irr=global, Pgrid=global, Qgrid=global, Qref=global, Vdc_mean=global, Vdc_ref=global
  wires:
  Rate Limiter/1 -> [Qref]
  (W/m2)/1 -> Manual Switch3/2
  (V)/1 -> Manual Switch2/2
  Steady-state Value4/1 -> Manual Switch/2
  DC Link Voltage Reference (Vdc_ref)/1 -> Manual Switch2/1
  System Fault Timing/1 -> Manual Switch/1
  Manual Switch/1 -> Rate Transition11/1
  Rate Limiter1/1 -> Rate Transition12/1
  (var)/1 -> Manual Switch1/2
  "Reactive Power Reference (Qref) "/1 -> Manual Switch1/1
  Manual Switch1/1 -> Rate Limiter/1
  Manual Switch2/1 -> [Vdc_ref]
  Irradiance (W/m2)/1 -> Manual Switch3/1
  Manual Switch3/1 -> Rate Limiter1/1
  Rate Transition12/1 -> [Irr]
  Bus Selector2/1 -> Rate Transition16/1  "<V_PV>"
  Bus Selector/2 -> Rate Transition15/1  "<I_PV>"
  Bus Selector/1 -> Rate Transition14/1  "<V_PV>"
  Rate Transition19/1 -> VIgrid/1  "Vabc"
  [Pm_PV1] -> Mux4/1  "Pmean PV1"
  Rate Transition17/1 -> PV Arrays voltages and currents/4  "Ipv2"
  RMS/1 -> Rate Transition22/1
  [Pm_PV2] -> Mux4/2  "Pmean PV2"
  [Irr] -> VP_PV12/1  "Irradiance"
  Rate Transition22/1 -> Vrms grid bus/1
  Rate Transition16/1 -> PV Arrays voltages and currents/3  "Vpv2"
  Rate Transition26/1 -> 25 kV bus/1  "Vabc"
  Mux3/1 -> VP_PV12/3
  [Vgrid] -> RMS/1
  [Vgrid] -> Power (Pos. Seq.)/1
  Rate Transition23/1 -> [Pgrid], PQgrid_MVA/1  "P (MW)"
  [PVArray1] -> Bus Selector/1
  Rate Transition20/1 -> VIgrid/2  "Iabc"
  Bus Selector1/2 -> Mux/2  "<Id>"
  Mux6/1 -> Vdcs/1
  Bus Selector1/1 -> Mux/1  "<Id_ref>"
  Mux4/1 -> VP_PV12/4
  Rate Transition15/1 -> PV Arrays voltages and currents/2  "Ipv1"
  Bus Selector1/3 -> Mux1/1  "<Iq_ref>"
  Mux5/1 -> VP_PV12/2
  Power (Pos. Seq.)/2 -> To-MW2/1
  [Igrid] -> Rate Transition20/1
  Rate Transition18/1 -> Fault current/1
  [Vabc25kV] -> Rate Transition26/1
  Mux1/1 -> Id & Iq/2
  Mux/1 -> Id & Iq/1
  Rate Transition25/1 -> 25 kV bus/2  "Iabc"
  Bus Selector3/2 -> Mux2/2  "<Qmeas>"
  [Vm_PV2] -> Mux3/2  "Vmean PV2"
  Rate Transition14/1 -> PV Arrays voltages and currents/1  "Vpv1"
  Mux2/1 -> Qs/1
  [Vgrid] -> Rate Transition19/1
  Rate Transition13/1 -> Mean/1, Mux6/2
  Power (Pos. Seq.)/1 -> To-KW/1
  [Dboost_PV1] -> Mux5/1  "D MPPT1"
  Bus Selector4/1 -> ModIndex/1  "<Mod Index>"
  Bus Selector3/1 -> Mux2/1  "<Qref>"
  [InverterControl] -> Bus Selector1/1, Bus Selector4/1, Bus Selector3/1
  [Vinv] -> Selector/1
  Mean/1 -> Mux6/3, [Vdc_mean]  "Vdc mean"
  Rate Transition11/1 -> [Fault]
  [Dboost_PV2] -> Mux5/2  "D MPPT2"
  [Vm_PV1] -> Mux3/1  "Vmean PV1"
  [Vdc_ref] -> Mux6/1  "Vdc_ref"
  Bus Selector1/4 -> Mux1/2  "<Iq>"
  [Igrid] -> Power (Pos. Seq.)/2
  Bus Selector2/2 -> Rate Transition17/1  "<I_PV>"
  [Iabc25kV] -> Rate Transition25/1
  Rate Transition24/1 -> [Qgrid], PQgrid_MVA/2  "Q (Mvar)"
  [Vdc] -> Rate Transition13/1
  [PVArray2] -> Bus Selector2/1
  [Ifault] -> Rate Transition18/1
  Selector/1 -> Rate Transition21/1
  Rate Transition21/1 -> Vab inverter bus/1
  To-MW2/1 -> Rate Transition24/1
  To-KW/1 -> Rate Transition23/1

== system PVFarmDistributionSystem/Subsystem ==

== system PVFarmDistributionSystem/Subsystem1 ==

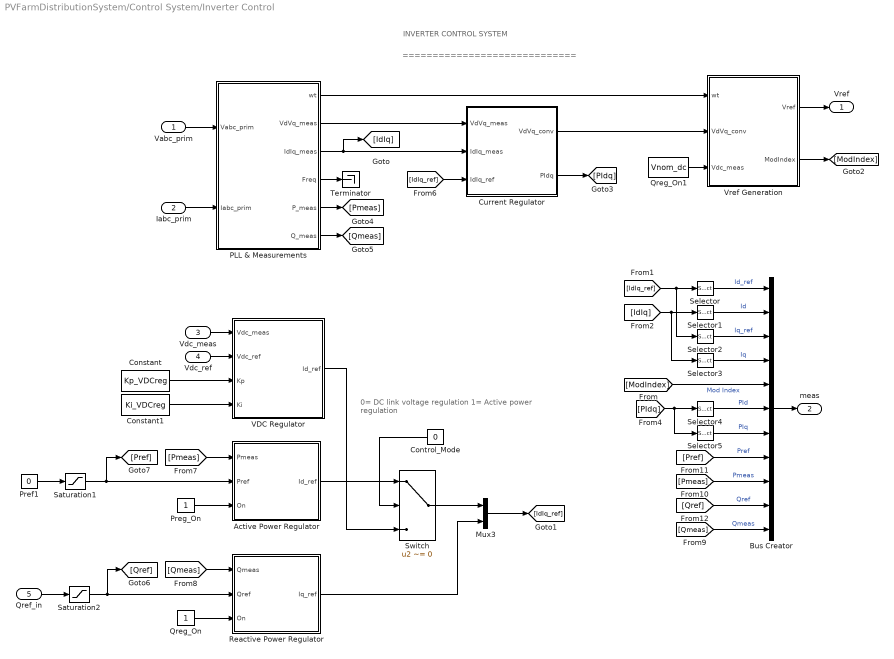
== system PVFarmDistributionSystem/Control System/Inverter Control ==
  note: INVERTER CONTROL SYSTEM
  note: =============================
  note: 0= DC link voltage regulation
      | 1= Active power regulation
  Vabc_prim : Inport  PortDimensions=3
  Iabc_prim : Inport  Port=2  PortDimensions=3
  Vdc_meas : Inport  Port=3  PortDimensions=1
  Vdc_ref : Inport  Port=4  PortDimensions=1
  Qref_in : Inport  Port=5  PortDimensions=1
  Active Power Regulator : Subsystem
  Bus Creator : BusCreator  Inputs=11
  Constant : Constant  Value=Kp_VDCreg  SampleTime=Ts
  Constant1 : Constant  Value=Ki_VDCreg  SampleTime=Ts
  Control_Mode : Constant  Value=0
  Current Regulator : Subsystem
  Mux3 : Mux  Inputs=2
  PLL & Measurements : Subsystem
  Pref1 : Constant  Value=0  SampleTime=Ts
  Preg_On : Constant
  Qreg_On : Constant
  Qreg_On1 : Constant  Value=Vnom_dc
  Reactive Power Regulator : Subsystem
  Saturation1 : Saturate  UpperLimit=2e6  LowerLimit=-2e6
  Saturation2 : Saturate  UpperLimit=1e6  LowerLimit=-1e6
  Selector : Selector  InputPortWidth=2  IndexOptions=Index vector (dialog)  Indices=1  OutputSizes=1
  Selector1 : Selector  InputPortWidth=2  IndexOptions=Index vector (dialog)  Indices=1  OutputSizes=1
  Selector2 : Selector  InputPortWidth=2  IndexOptions=Index vector (dialog)  Indices=2  OutputSizes=1
  Selector3 : Selector  InputPortWidth=2  IndexOptions=Index vector (dialog)  Indices=2  OutputSizes=1
  Selector4 : Selector  InputPortWidth=2  IndexOptions=Index vector (dialog)  Indices=1  OutputSizes=1
  Selector5 : Selector  InputPortWidth=2  IndexOptions=Index vector (dialog)  Indices=2  OutputSizes=1
  Switch : Switch  Criteria=u2 ~= 0  SaturateOnIntegerOverflow=off  InputSameDT=off
  Terminator : Terminator
  VDC Regulator : Subsystem
  Vref Generation : Subsystem
  Vref : Outport  VectorParamsAs1DForOutWhenUnconnected=off
  meas : Outport  Port=2  VectorParamsAs1DForOutWhenUnconnected=off
  wires:
  Constant/1 -> VDC Regulator/3(Kp)
  Control_Mode/1 -> Switch/2
  Active Power Regulator/1(Id_ref) -> Switch/1
  VDC Regulator/1(Id_ref) -> Switch/3
  Current Regulator/1(VdVq_conv) -> Vref Generation/2(VdVq_conv)
  Qreg_On/1 -> Reactive Power Regulator/3(On)
  PLL & Measurements/1(wt) -> Vref Generation/1(wt)
  Selector3/1 -> Bus Creator/4  "Iq"
  PLL & Measurements/2(VdVq_meas) -> Current Regulator/1(VdVq_meas)
  [ModIndex] -> Bus Creator/5  "Mod Index"
  [IdIq_ref] -> Selector/1, Selector2/1
  Pref1/1 -> Saturation1/1
  PLL & Measurements/5(P_meas) -> [Pmeas]
  Current Regulator/2(PIdq) -> [PIdq]
  Vabc_prim/1 -> PLL & Measurements/1(Vabc_prim)
  Mux3/1 -> [IdIq_ref]
  [Pmeas] -> Bus Creator/9  "Pmeas"
  Reactive Power Regulator/1(Iq_ref) -> Mux3/2
  [PIdq] -> Selector5/1, Selector4/1
  [IdIq_ref] -> Current Regulator/3(IdIq_ref)
  [Qmeas] -> Reactive Power Regulator/1(Qmeas)
  PLL & Measurements/6(Q_meas) -> [Qmeas]
  Selector2/1 -> Bus Creator/3  "Iq_ref"
  [Pmeas] -> Active Power Regulator/1(Pmeas)
  [Qref] -> Bus Creator/10  "Qref"
  [Pref] -> Bus Creator/8  "Pref"
  Selector/1 -> Bus Creator/1  "Id_ref"
  [Qmeas] -> Bus Creator/11  "Qmeas"
  PLL & Measurements/3(IdIq_meas) -> Current Regulator/2(IdIq_meas), [IdIq]
  Vdc_ref/1 -> VDC Regulator/2(Vdc_ref)
  [IdIq] -> Selector1/1, Selector3/1
  Preg_On/1 -> Active Power Regulator/3(On)
  Switch/1 -> Mux3/1
  Vref Generation/2(ModIndex) -> [ModIndex]
  Iabc_prim/1 -> PLL & Measurements/2(Iabc_prim)
  PLL & Measurements/4(Freq) -> Terminator/1
  Vref Generation/1(Vref) -> Vref/1
  Selector4/1 -> Bus Creator/6  "PId"
  Vdc_meas/1 -> VDC Regulator/1(Vdc_meas)
  Selector5/1 -> Bus Creator/7  "PIq"
  Selector1/1 -> Bus Creator/2  "Id"
  Qreg_On1/1 -> Vref Generation/3(Vdc_meas)
  Qref_in/1 -> Saturation2/1
  Saturation2/1 -> [Qref], Reactive Power Regulator/2(Qref)
  Constant1/1 -> VDC Regulator/4(Ki)
  Bus Creator/1 -> meas/1
  Saturation1/1 -> [Pref], Active Power Regulator/2(Pref)

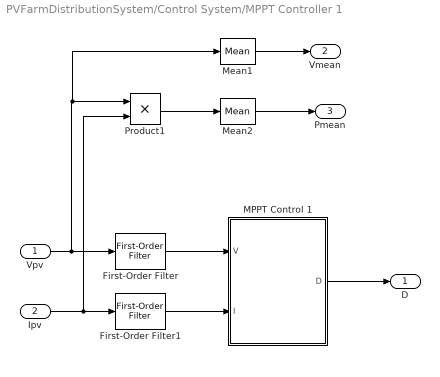
== system PVFarmDistributionSystem/Control System/MPPT Controller 1 ==
  Vpv : Inport
  Ipv : Inport  Port=2
  First-Order Filter : spsFirstOrderFilterLib/First-Order Filter  FilterType=Lowpass  Tc=1/Fc  Ts=Ts  Initialize=off  Vac_Init=[0, 0, 60]  Vdc_Init=0  PlotResponse=off  FreqRange="[0,  200,  1]"
  First-Order Filter1 : spsFirstOrderFilterLib/First-Order Filter  FilterType=Lowpass  Tc=1/Fc  Ts=Ts  Initialize=off  Vac_Init=[0, 0, 60]  Vdc_Init=0  PlotResponse=off  FreqRange="[0,  200,  1]"
  "MPPT Control 1 " : MATLAB Function  TreatAsAtomicUnit=on
  Mean1 : spsMeanLib/Mean  Freq=60  Vinit=650  Ts=Ts
  Mean2 : spsMeanLib/Mean  Freq=60  Vinit=1500e3  Ts=Ts
  Product1 : Product
  D : Outport  VectorParamsAs1DForOutWhenUnconnected=off
  Vmean : Outport  Port=2  VectorParamsAs1DForOutWhenUnconnected=off
  Pmean : Outport  Port=3  VectorParamsAs1DForOutWhenUnconnected=off
  wires:
  First-Order Filter1/1 -> "MPPT Control 1 "/2(I)
  First-Order Filter/1 -> "MPPT Control 1 "/1(V)
  Ipv/1 -> Product1/2, First-Order Filter1/1
  Vpv/1 -> Mean1/1, Product1/1, First-Order Filter/1
  "MPPT Control 1 "/1(D) -> D/1
  Product1/1 -> Mean2/1
  Mean1/1 -> Vmean/1
  Mean2/1 -> Pmean/1

== system PVFarmDistributionSystem/Control System/MPPT Controller 2 ==
  Vpv : Inport
  Ipv : Inport  Port=2
  First-Order Filter : spsFirstOrderFilterLib/First-Order Filter  FilterType=Lowpass  Tc=1/Fc  Ts=Ts  Initialize=off  Vac_Init=[0, 0, 60]  Vdc_Init=0  PlotResponse=off  FreqRange="[0,  200,  1]"
  First-Order Filter1 : spsFirstOrderFilterLib/First-Order Filter  FilterType=Lowpass  Tc=1/Fc  Ts=Ts  Initialize=off  Vac_Init=[0, 0, 60]  Vdc_Init=0  PlotResponse=off  FreqRange="[0,  200,  1]"
  "MPPT Control 1 " : MATLAB Function  TreatAsAtomicUnit=on
  Mean1 : spsMeanLib/Mean  Freq=60  Vinit=420  Ts=Ts
  Mean2 : spsMeanLib/Mean  Freq=60  Vinit=500e3  Ts=Ts
  Product1 : Product
  D : Outport  VectorParamsAs1DForOutWhenUnconnected=off
  Vmean : Outport  Port=2  VectorParamsAs1DForOutWhenUnconnected=off
  Pmean : Outport  Port=3  VectorParamsAs1DForOutWhenUnconnected=off
  wires:
  "MPPT Control 1 "/1(D) -> D/1
  Ipv/1 -> Product1/2, First-Order Filter1/1
  First-Order Filter/1 -> "MPPT Control 1 "/1(V)
  First-Order Filter1/1 -> "MPPT Control 1 "/2(I)
  Mean1/1 -> Vmean/1
  Product1/1 -> Mean2/1
  Mean2/1 -> Pmean/1
  Vpv/1 -> Product1/1, Mean1/1, First-Order Filter/1
